simulink library "OpenSCENARIO"  (R2019a)
settings: Solver=VariableStepAuto  StartTime=0.0  StopTime=10.0  RelTol=1e-3
undefined symbols (not defined in the file or in its folder): A1, car, DiscIntNeverNeededParam, i, t1, W1
libraries: adeye_lib x6, $bdroot x2, simulink x2
settings Model: Creator=adeye  LastModifiedBy=adeye

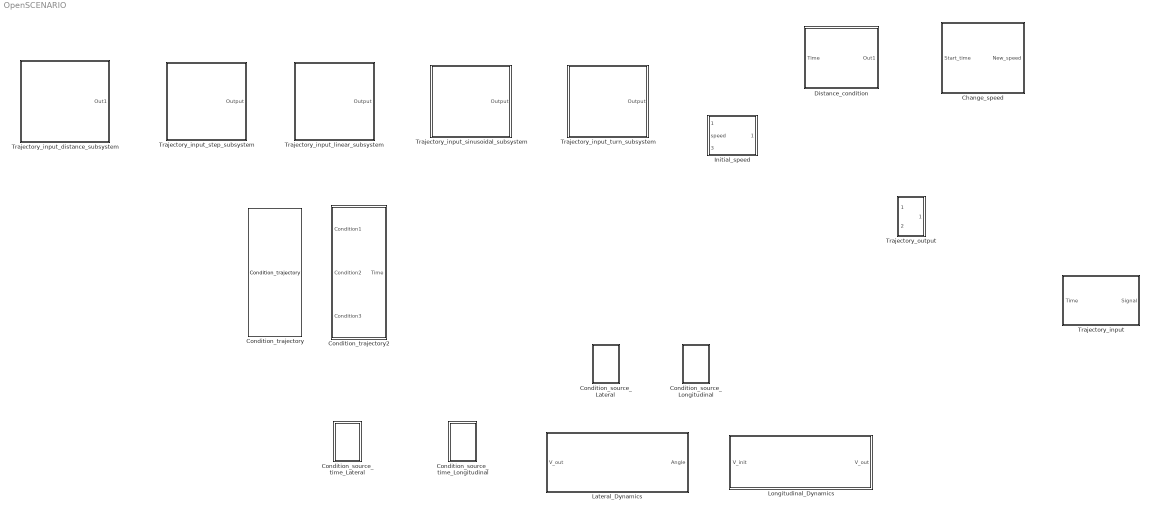
== system OpenSCENARIO ==
  Change_speed : Subsystem
  Condition_source_Lateral : Subsystem
  Condition_source_Longitudinal : Subsystem
  Condition_source_time_Lateral : Subsystem
  Condition_source_time_Longitudinal : Subsystem
  Condition_trajectory : $bdroot/Trajectory_input_step_subsystem/Condition_trajectory  SystemSampleTime=-1
      link override Gain2: Gain=1
      link override Switch1: Threshold=0.001
  Condition_trajectory2 : Subsystem
  Distance_condition : Subsystem
  Initial_speed : Subsystem
  Lateral_Dynamics : Subsystem
  Longitudinal_Dynamics : Subsystem
  Trajectory_input : Subsystem
  Trajectory_input_distance_subsystem : Subsystem
  Trajectory_input_linear_subsystem : Subsystem
  Trajectory_input_sinusoidal_subsystem : Subsystem
  Trajectory_input_step_subsystem : Subsystem
  Trajectory_input_turn_subsystem : Subsystem  AncestorBlock=OpenSCENARIO/Trajectory_input_sinusoidal_subsystem
  Trajectory_output : Subsystem

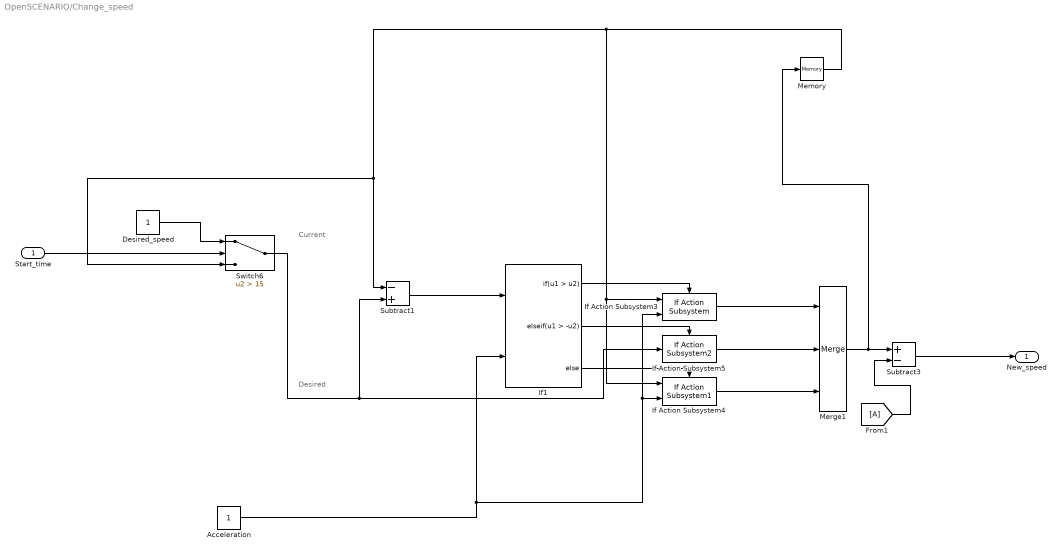
== system OpenSCENARIO/Change_speed ==
  note: Current
  note: Desired
  Start_time : Inport
  Acceleration : Constant
  Desired_speed : Constant
  If Action Subsystem3 : adeye_lib/Subsystem1/Subsystem/If Action Subsystem  SystemSampleTime=-1
  If Action Subsystem4 : adeye_lib/Subsystem1/Subsystem/If Action Subsystem1  SystemSampleTime=-1
  If Action Subsystem5 : adeye_lib/Subsystem1/Subsystem/If Action Subsystem2  SystemSampleTime=-1
  If1 : If  NumInputs=2  IfExpression=u1 > u2  ElseIfExpressions=u1 > -u2
  Memory : Memory  InitialCondition=-5/3.6
  Merge1 : Merge  Inputs=3
  Subtract1 : Sum  Inputs=-+
  Subtract3 : Sum  Inputs=+-
  Switch6 : Switch  Criteria=u2 > Threshold  Threshold=15
  "New_speed " : Outport
  wires:
  If Action Subsystem3/1 -> Merge1/1
  If Action Subsystem4/1 -> Merge1/3
  If1/1 -> If Action Subsystem3/Action
  Start_time/1 -> Switch6/2
  If Action Subsystem5/1 -> Merge1/2
  Acceleration/1 -> If1/2, If Action Subsystem4/2, If Action Subsystem3/2
  If1/3 -> If Action Subsystem4/Action
  If1/2 -> If Action Subsystem5/Action
  Desired_speed/1 -> Switch6/1
  Switch6/1 -> Subtract1/2, If Action Subsystem5/1
  Subtract1/1 -> If1/1
  Merge1/1 -> Memory/1, Subtract3/1
  [A] -> Subtract3/2
  Subtract3/1 -> "New_speed "/1
  Memory/1 -> If Action Subsystem3/1, If Action Subsystem4/1, Switch6/3, Subtract1/1

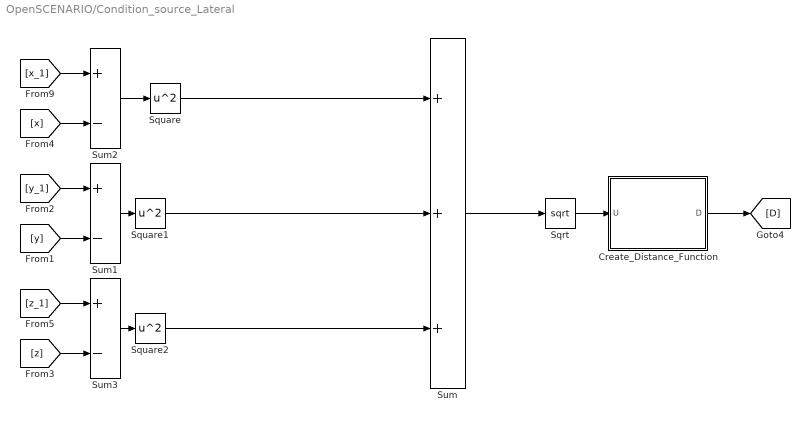
== system OpenSCENARIO/Condition_source_Lateral ==
  Create_Distance_Function : Subsystem
  Sqrt : Sqrt  SaturateOnIntegerOverflow=on
  Square : Math  Operator=square  SaturateOnIntegerOverflow=on
  Square1 : Math  Operator=square  SaturateOnIntegerOverflow=on
  Square2 : Math  Operator=square  SaturateOnIntegerOverflow=on
  Sum : Sum  Inputs=+++
  Sum1 : Sum  Inputs=+-
  Sum2 : Sum  Inputs=+-
  Sum3 : Sum  Inputs=+-
  wires:
  [x_1] -> Sum2/1
  [x] -> Sum2/2
  [y_1] -> Sum1/1
  [y] -> Sum1/2
  [z] -> Sum3/2
  [z_1] -> Sum3/1
  Sum/1 -> Sqrt/1
  Sum1/1 -> Square1/1
  Sum2/1 -> Square/1
  Square1/1 -> Sum/2
  Sum3/1 -> Square2/1
  Square2/1 -> Sum/3
  Square/1 -> Sum/1
  Create_Distance_Function/1(D) -> [D]
  Sqrt/1 -> Create_Distance_Function/1(U)

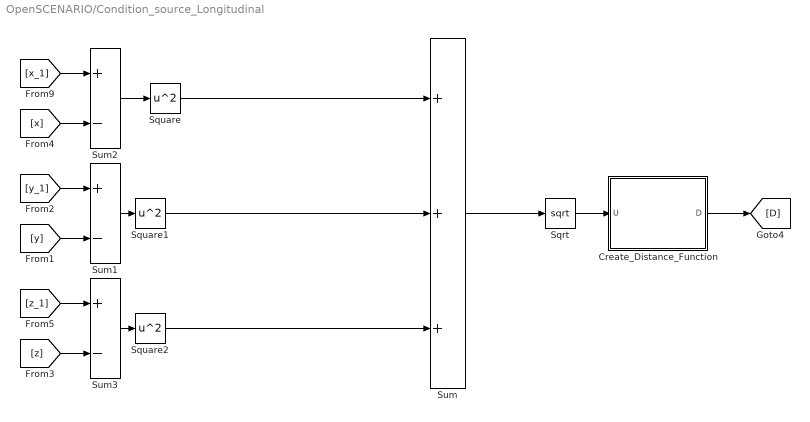
== system OpenSCENARIO/Condition_source_Longitudinal ==
  Create_Distance_Function : Subsystem
  Sqrt : Sqrt  SaturateOnIntegerOverflow=on
  Square : Math  Operator=square  SaturateOnIntegerOverflow=on
  Square1 : Math  Operator=square  SaturateOnIntegerOverflow=on
  Square2 : Math  Operator=square  SaturateOnIntegerOverflow=on
  Sum : Sum  Inputs=+++
  Sum1 : Sum  Inputs=+-
  Sum2 : Sum  Inputs=+-
  Sum3 : Sum  Inputs=+-
  wires:
  [x_1] -> Sum2/1
  [x] -> Sum2/2
  [y_1] -> Sum1/1
  [y] -> Sum1/2
  [z] -> Sum3/2
  [z_1] -> Sum3/1
  Sum/1 -> Sqrt/1
  Sum1/1 -> Square1/1
  Sum2/1 -> Square/1
  Square1/1 -> Sum/2
  Sum3/1 -> Square2/1
  Square2/1 -> Sum/3
  Square/1 -> Sum/1
  Create_Distance_Function/1(D) -> [D]
  Sqrt/1 -> Create_Distance_Function/1(U)

== system OpenSCENARIO/Condition_source_time_Lateral ==
  Constant : Constant
  Integrator : Integrator
  wires:
  Constant/1 -> Integrator/1
  Integrator/1 -> [D]

== system OpenSCENARIO/Condition_source_time_Longitudinal ==
  Constant : Constant
  Integrator : Integrator
  wires:
  Constant/1 -> Integrator/1
  Integrator/1 -> [D]

== system OpenSCENARIO/Condition_trajectory2 ==
  Condition1 : Inport
  Condition2 : Inport  Port=2
  Condition3 : Inport  Port=3
  Constant1 : Constant  Value=0
  Integrator1 : Integrator
  Rounding Function : Rounding
  Scope4 : Scope
  Switch1 : Switch  Criteria=u2 > Threshold  Threshold=-str2double(car(2).trajectory(1,i).condition.general.value)
  Variable Integer Delay : Delay  DelayLengthSource=Input port
      settings: InputPortMap=u0,p1
  Time : Outport
  wires:
  Switch1/1 -> Integrator1/1
  Condition2/1 -> Switch1/2
  Integrator1/1 -> Variable Integer Delay/1
  Variable Integer Delay/1 -> Scope4/1, Time/1
  Constant1/1 -> Rounding Function/1
  Rounding Function/1 -> Variable Integer Delay/2
  Condition1/1 -> Switch1/1
  Condition3/1 -> Switch1/3

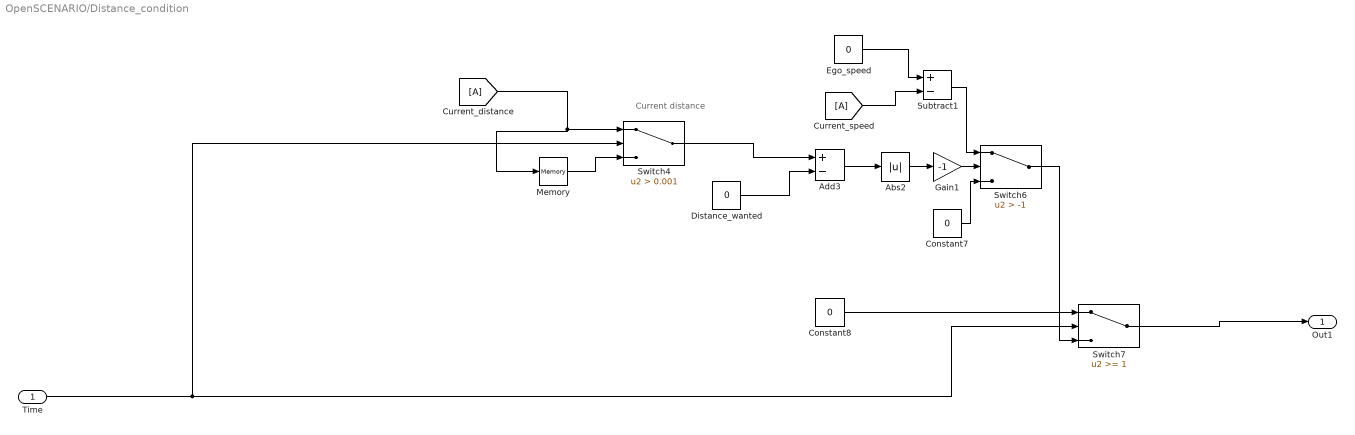
== system OpenSCENARIO/Distance_condition ==
  note: Current distance
  Time : Inport
  Abs2 : Abs  OutDataTypeStr=Inherit: Inherit via internal rule
  Add3 : Sum  Inputs=+-
  Constant7 : Constant  Value=0
  Constant8 : Constant  Value=0
  Distance_wanted : Constant  Value=0
  Ego_speed : Constant  Value=0
  Gain1 : Gain  Gain=-1
  Memory : Memory
  Subtract1 : Sum  Inputs=+-
  Switch4 : Switch  Criteria=u2 > Threshold  Threshold=0.001
  Switch6 : Switch  Criteria=u2 > Threshold  Threshold=-1
  Switch7 : Switch  Threshold=1
  Out1 : Outport
  wires:
  Gain1/1 -> Switch6/2
  Abs2/1 -> Gain1/1
  Switch7/1 -> Out1/1
  Constant8/1 -> Switch7/1
  Time/1 -> Switch4/2, Switch7/2
  Switch4/1 -> Add3/1
  [A] -> Subtract1/2
  Switch6/1 -> Switch7/3
  Constant7/1 -> Switch6/3
  Subtract1/1 -> Switch6/1
  Distance_wanted/1 -> Add3/2
  Ego_speed/1 -> Subtract1/1
  Add3/1 -> Abs2/1
  Memory/1 -> Switch4/3
  [A] -> Memory/1, Switch4/1

== system OpenSCENARIO/Initial_speed ==
  Initial_speed : Inport
  speed : Inport  Port=2
  Step_time : Inport  Port=3
  Clock : Clock
  If : If  NumInputs=2  IfExpression=u1 < u2
  If Action Subsystem : Subsystem  TreatAsAtomicUnit=on
  If Action Subsystem1 : Subsystem  TreatAsAtomicUnit=on
  Merge : Merge
  ego_speed : Outport
  wires:
  Initial_speed/1 -> If Action Subsystem/1(In1)
  Merge/1 -> ego_speed/1
  Clock/1 -> If/1
  If/1 -> If Action Subsystem/Action
  speed/1 -> If Action Subsystem1/1(In1)
  If/2 -> If Action Subsystem1/Action
  If Action Subsystem/1(Out1) -> Merge/1
  If Action Subsystem1/1(Out1) -> Merge/2
  Step_time/1 -> If/2

== system OpenSCENARIO/Lateral_Dynamics ==
  V_out : Inport
  Add : Sum
  Trajectory_output : Subsystem
  Angle : Outport
  tag scope: V_out=global
  wires:
  Trajectory_output/1(Angle) -> Angle/1
  Add/1 -> Trajectory_output/2(Signal)
  V_out/1 -> [V_out], Trajectory_output/1(V_init)

== system OpenSCENARIO/Longitudinal_Dynamics ==
  V_init : Inport
  Add : Sum
  V_out : Outport
  tag scope: V_in=global
  wires:
  Add/1 -> V_out/1
  V_init/1 -> [V_in], Add/1

== system OpenSCENARIO/Trajectory_input ==
  Time : Inport
  Constant3 : Constant  Value=A1
  Gain4 : Gain  Gain=-1
  Gain5 : Gain  Gain=A1
  Gain6 : Gain  Gain=W1
  Memory : Memory
  Sine1 : Trigonometry
  Switch3 : Switch  Criteria=u2 > Threshold  Threshold=-t1
  Signal : Outport
  wires:
  Time/1 -> Gain5/1, Gain4/1, Gain6/1
  Gain6/1 -> Sine1/1
  Gain4/1 -> Switch3/2
  Switch3/1 -> Memory/1, Signal/1
  Gain5/1 -> Switch3/1
  Memory/1 -> Switch3/3

== system OpenSCENARIO/Trajectory_input_distance_subsystem ==
  Condition_trajectory : $bdroot/Trajectory_input_step_subsystem/Condition_trajectory  SystemSampleTime=-1
      link override Gain2: Gain=1
      link override Switch1: Threshold=0.001
      link override Switch2: Threshold=0  Criteria=u2 >= Threshold
  Distance_condition : Subsystem  AncestorBlock=OpenSCENARIO/Distance_condition
  Out1 : Outport
  wires:
  Condition_trajectory/1 -> Distance_condition/1(Time)
  Distance_condition/1(Out1) -> Out1/1

== system OpenSCENARIO/Trajectory_input_linear_subsystem ==
  Change_speed : Subsystem  AncestorBlock=OpenSCENARIO/Change_speed
  Condition_trajectory : Subsystem
  Output : Outport
  wires:
  Change_speed/1("New_speed ") -> Output/1
  Condition_trajectory/1(Time) -> Change_speed/1(Start_time)

== system OpenSCENARIO/Trajectory_input_sinusoidal_subsystem ==
  Condition_trajectory : Subsystem
  Trajectory_input : Subsystem
  Output : Outport
  wires:
  Condition_trajectory/1(Time) -> Trajectory_input/1(Time)
  Trajectory_input/1(Signal) -> Output/1

== system OpenSCENARIO/Trajectory_input_step_subsystem ==
  Condition_trajectory : Subsystem
  Trajectory_input : Subsystem
  Output : Outport
  wires:
  Condition_trajectory/1(Time) -> Trajectory_input/1(Time)
  Trajectory_input/1(Signal) -> Output/1

== system OpenSCENARIO/Trajectory_input_turn_subsystem ==
  Condition_trajectory : Subsystem
  Trajectory_input : Subsystem
  Output : Outport
  wires:
  Condition_trajectory/1(Time) -> Trajectory_input/1(Time)
  Trajectory_input/1(Signal) -> Output/1

== system OpenSCENARIO/Trajectory_output ==
  V_init : Inport
  Signal : Inport  Port=2
  Asin : Trigonometry  Operator=asin
  Discrete Derivative : simulink/Discrete/Discrete Derivative  gainval=1.0  ICPrevScaledInput=0.0  OutMin=[]  OutMax=[]  OutDataType=fixdt(1, 16)  OutScaling=2^-10  DoSatur=off
  Divide : Product  Inputs=/*
  Angle : Outport
  wires:
  Divide/1 -> Asin/1
  Discrete Derivative/1 -> Divide/2
  Signal/1 -> Discrete Derivative/1
  V_init/1 -> Divide/1
  Asin/1 -> Angle/1

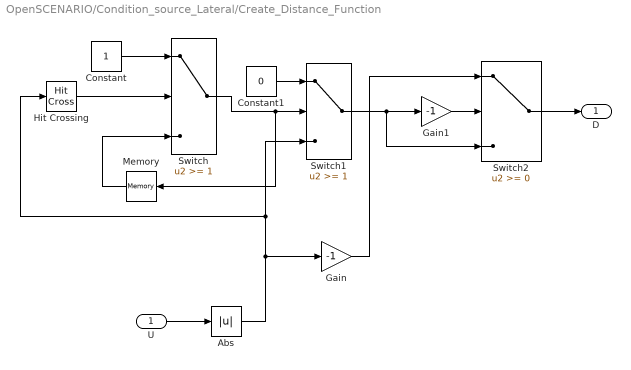
== system OpenSCENARIO/Condition_source_Lateral/Create_Distance_Function ==
  U : Inport
  Abs : Abs
  Constant : Constant
  Constant1 : Constant  Value=0
  Gain : Gain  Gain=-1
  Gain1 : Gain  Gain=-1
  Hit Crossing : HitCross  HitCrossingOffset=0.5
  Memory : Memory
  Switch : Switch  Threshold=1
  Switch1 : Switch  Threshold=1
  Switch2 : Switch
  D : Outport
  wires:
  Abs/1 -> Switch1/3, Hit Crossing/1, Gain/1
  Constant1/1 -> Switch1/1
  Memory/1 -> Switch/3
  Switch/1 -> Memory/1, Switch1/2
  Gain1/1 -> Switch2/2
  Hit Crossing/1 -> Switch/2
  Switch1/1 -> Switch2/3, Gain1/1
  Switch2/1 -> D/1
  Gain/1 -> Switch2/1
  Constant/1 -> Switch/1
  U/1 -> Abs/1

== system OpenSCENARIO/Condition_source_Longitudinal/Create_Distance_Function ==
  U : Inport
  Abs : Abs
  Constant : Constant
  Constant1 : Constant  Value=0
  Gain : Gain  Gain=-1
  Gain1 : Gain  Gain=-1
  Hit Crossing : HitCross  HitCrossingOffset=0.5
  Memory : Memory
  Switch : Switch  Threshold=1
  Switch1 : Switch  Threshold=1
  Switch2 : Switch
  D : Outport
  wires:
  Abs/1 -> Switch1/3, Hit Crossing/1, Gain/1
  Constant1/1 -> Switch1/1
  Memory/1 -> Switch/3
  Switch/1 -> Memory/1, Switch1/2
  Gain1/1 -> Switch2/2
  Hit Crossing/1 -> Switch/2
  Switch1/1 -> Switch2/3, Gain1/1
  Switch2/1 -> D/1
  Gain/1 -> Switch2/1
  Constant/1 -> Switch/1
  U/1 -> Abs/1

== system OpenSCENARIO/Initial_speed/If Action Subsystem ==
  In1 : Inport
  Action Port : ActionPort
  Out1 : Outport
  wires:
  In1/1 -> Out1/1

== system OpenSCENARIO/Initial_speed/If Action Subsystem1 ==
  In1 : Inport
  Action Port : ActionPort
  Out1 : Outport
  wires:
  In1/1 -> Out1/1

== system OpenSCENARIO/Lateral_Dynamics/Trajectory_output ==
  V_init : Inport
  Signal : Inport  Port=2
  Asin : Trigonometry  Operator=asin
  Constant : Constant
  Discrete Derivative : simulink/Discrete/Discrete Derivative  gainval=1.0  ICPrevScaledInput=0.0  OutMin=[]  OutMax=[]  OutDataType=fixdt(1, 16)  OutScaling=2^-10  DoSatur=off
  Divide : Product  Inputs=/*
  Switch : Switch  Criteria=u2 > Threshold
  Angle : Outport
  wires:
  Divide/1 -> Asin/1
  Discrete Derivative/1 -> Divide/2
  Signal/1 -> Discrete Derivative/1
  V_init/1 -> Divide/1
  Switch/1 -> Angle/1
  Asin/1 -> Switch/1
  [W] -> Switch/2
  Constant/1 -> Switch/3

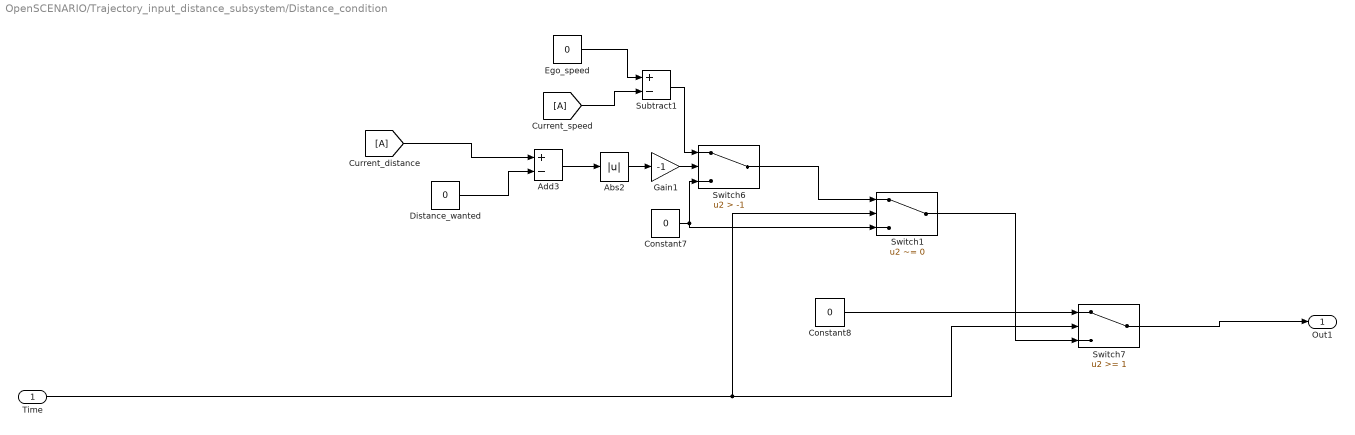
== system OpenSCENARIO/Trajectory_input_distance_subsystem/Distance_condition ==
  Time : Inport
  Abs2 : Abs  OutDataTypeStr=Inherit: Inherit via internal rule
  Add3 : Sum  Inputs=+-
  Constant7 : Constant  Value=0
  Constant8 : Constant  Value=0
  Distance_wanted : Constant  Value=0
  Ego_speed : Constant  Value=0
  Gain1 : Gain  Gain=-1
  Subtract1 : Sum  Inputs=+-
  Switch1 : Switch  Criteria=u2 ~= 0  Threshold=-1
  Switch6 : Switch  Criteria=u2 > Threshold  Threshold=-1
  Switch7 : Switch  Threshold=1
  Out1 : Outport
  wires:
  Gain1/1 -> Switch6/2
  Abs2/1 -> Gain1/1
  Switch7/1 -> Out1/1
  Constant8/1 -> Switch7/1
  Time/1 -> Switch1/2, Switch7/2
  [A] -> Add3/1
  [A] -> Subtract1/2
  Constant7/1 -> Switch6/3, Switch1/3
  Subtract1/1 -> Switch6/1
  Distance_wanted/1 -> Add3/2
  Ego_speed/1 -> Subtract1/1
  Add3/1 -> Abs2/1
  Switch1/1 -> Switch7/3
  Switch6/1 -> Switch1/1

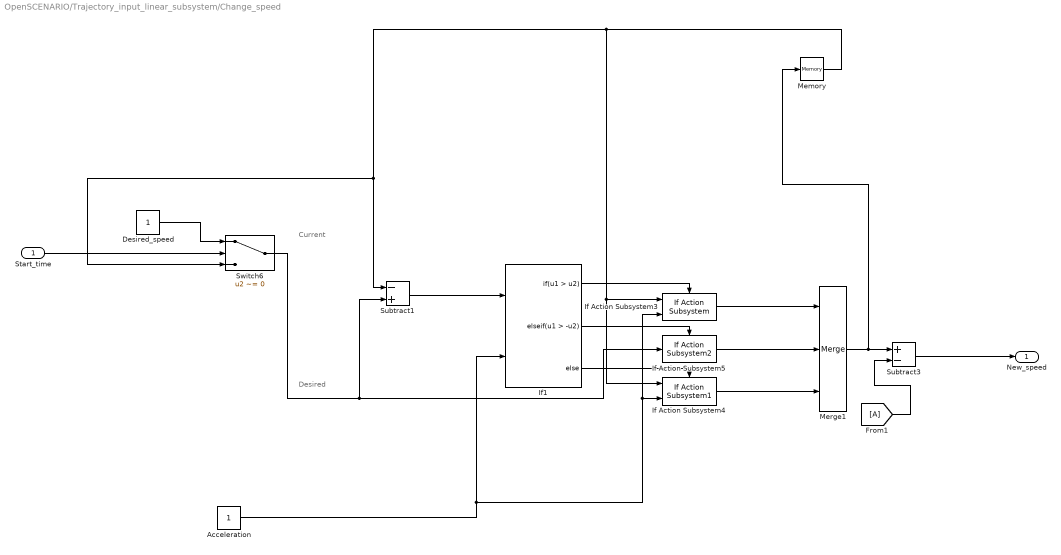
== system OpenSCENARIO/Trajectory_input_linear_subsystem/Change_speed ==
  note: Desired
  note: Current
  Start_time : Inport
  Acceleration : Constant
  Desired_speed : Constant
  If Action Subsystem3 : adeye_lib/Subsystem1/Subsystem/If Action Subsystem  SystemSampleTime=-1
  If Action Subsystem4 : adeye_lib/Subsystem1/Subsystem/If Action Subsystem1  SystemSampleTime=-1
  If Action Subsystem5 : adeye_lib/Subsystem1/Subsystem/If Action Subsystem2  SystemSampleTime=-1
  If1 : If  NumInputs=2  IfExpression=u1 > u2  ElseIfExpressions=u1 > -u2
  Memory : Memory  InitialCondition=-5/3.6
  Merge1 : Merge  Inputs=3
  Subtract1 : Sum  Inputs=-+
  Subtract3 : Sum  Inputs=+-
  Switch6 : Switch  Criteria=u2 ~= 0  Threshold=15
  "New_speed " : Outport
  wires:
  Memory/1 -> Subtract1/1, Switch6/3, If Action Subsystem4/1, If Action Subsystem3/1
  Subtract3/1 -> "New_speed "/1
  [A] -> Subtract3/2
  Merge1/1 -> Subtract3/1, Memory/1
  Subtract1/1 -> If1/1
  Switch6/1 -> If Action Subsystem5/1, Subtract1/2
  Desired_speed/1 -> Switch6/1
  If1/2 -> If Action Subsystem5/Action
  If1/3 -> If Action Subsystem4/Action
  Acceleration/1 -> If Action Subsystem3/2, If Action Subsystem4/2, If1/2
  If Action Subsystem5/1 -> Merge1/2
  Start_time/1 -> Switch6/2
  If1/1 -> If Action Subsystem3/Action
  If Action Subsystem4/1 -> Merge1/3
  If Action Subsystem3/1 -> Merge1/1

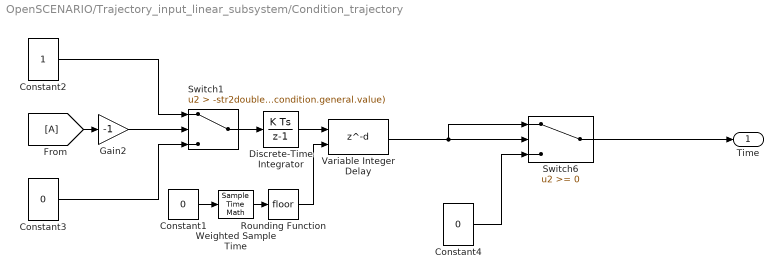
== system OpenSCENARIO/Trajectory_input_linear_subsystem/Condition_trajectory ==
  Constant1 : Constant  Value=0
  Constant2 : Constant
  Constant3 : Constant  Value=0
  Constant4 : Constant  Value=0
  Discrete-Time Integrator : DiscreteIntegrator  SampleTime=-1  ICPrevOutput=DiscIntNeverNeededParam  ICPrevScaledInput=DiscIntNeverNeededParam
  Gain2 : Gain  Gain=-1
  Rounding Function : Rounding
  Switch1 : Switch  Criteria=u2 > Threshold  Threshold=-str2double(car(2).trajectory(1,i).condition.general.value)
  Switch6 : Switch
  Variable Integer Delay : Delay  DelayLengthSource=Input port  DelayLengthUpperLimit=999
      settings: InputPortMap=u0,p1
  Weighted Sample Time : SampleTimeMath  TsampMathOp=/  TsampMathImp=Offline Scaling Adjustment
  Time : Outport
  wires:
  Rounding Function/1 -> Variable Integer Delay/2
  Constant1/1 -> Weighted Sample Time/1
  Discrete-Time Integrator/1 -> Variable Integer Delay/1
  Gain2/1 -> Switch1/2
  Switch1/1 -> Discrete-Time Integrator/1
  Constant3/1 -> Switch1/3
  Constant2/1 -> Switch1/1
  [A] -> Gain2/1
  Weighted Sample Time/1 -> Rounding Function/1
  Switch6/1 -> Time/1
  Variable Integer Delay/1 -> Switch6/1, Switch6/2
  Constant4/1 -> Switch6/3

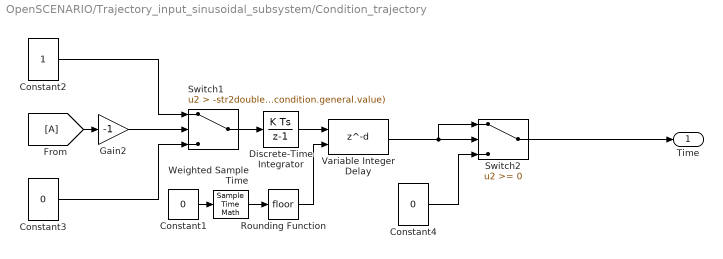
== system OpenSCENARIO/Trajectory_input_sinusoidal_subsystem/Condition_trajectory ==
  Constant1 : Constant  Value=0
  Constant2 : Constant
  Constant3 : Constant  Value=0
  Constant4 : Constant  Value=0
  Discrete-Time Integrator : DiscreteIntegrator  SampleTime=-1  ICPrevOutput=DiscIntNeverNeededParam  ICPrevScaledInput=DiscIntNeverNeededParam
  Gain2 : Gain  Gain=-1
  Rounding Function : Rounding
  Switch1 : Switch  Criteria=u2 > Threshold  Threshold=-str2double(car(2).trajectory(1,i).condition.general.value)
  Switch2 : Switch
  Variable Integer Delay : Delay  DelayLengthSource=Input port  DelayLengthUpperLimit=999
      settings: InputPortMap=u0,p1
  Weighted Sample Time : SampleTimeMath  TsampMathOp=/  TsampMathImp=Offline Scaling Adjustment
  Time : Outport
  wires:
  Rounding Function/1 -> Variable Integer Delay/2
  Discrete-Time Integrator/1 -> Variable Integer Delay/1
  Gain2/1 -> Switch1/2
  Switch1/1 -> Discrete-Time Integrator/1
  Constant3/1 -> Switch1/3
  Constant2/1 -> Switch1/1
  [A] -> Gain2/1
  Constant1/1 -> Weighted Sample Time/1
  Weighted Sample Time/1 -> Rounding Function/1
  Switch2/1 -> Time/1
  Variable Integer Delay/1 -> Switch2/1, Switch2/2
  Constant4/1 -> Switch2/3

== system OpenSCENARIO/Trajectory_input_sinusoidal_subsystem/Trajectory_input ==
  Time : Inport
  Constant3 : Constant  Value=A1
  Cos : Trigonometry  Operator=cos
  Gain4 : Gain  Gain=-1
  Gain5 : Gain  Gain=A1
  Gain6 : Gain  Gain=W1
  Switch3 : Switch  Criteria=u2 > Threshold  Threshold=-t1
  Signal : Outport
  tag scope: W=global
  wires:
  Gain5/1 -> Switch3/1
  Constant3/1 -> Switch3/3
  Time/1 -> Gain4/1, Gain6/1
  Gain6/1 -> Cos/1
  Gain4/1 -> [W], Switch3/2
  Cos/1 -> Gain5/1
  Switch3/1 -> Signal/1

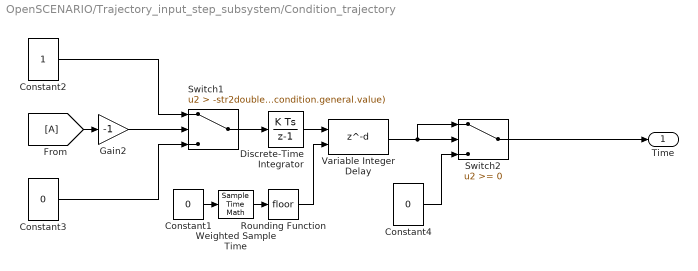
== system OpenSCENARIO/Trajectory_input_step_subsystem/Condition_trajectory ==
  Constant1 : Constant  Value=0
  Constant2 : Constant
  Constant3 : Constant  Value=0
  Constant4 : Constant  Value=0
  Discrete-Time Integrator : DiscreteIntegrator  SampleTime=-1  ICPrevOutput=DiscIntNeverNeededParam  ICPrevScaledInput=DiscIntNeverNeededParam
  Gain2 : Gain  Gain=-1
  Rounding Function : Rounding
  Switch1 : Switch  Criteria=u2 > Threshold  Threshold=-str2double(car(2).trajectory(1,i).condition.general.value)
  Switch2 : Switch
  Variable Integer Delay : Delay  DelayLengthSource=Input port  DelayLengthUpperLimit=999
      settings: InputPortMap=u0,p1
  Weighted Sample Time : SampleTimeMath  TsampMathOp=/  TsampMathImp=Offline Scaling Adjustment
  Time : Outport
  wires:
  Rounding Function/1 -> Variable Integer Delay/2
  Discrete-Time Integrator/1 -> Variable Integer Delay/1
  Gain2/1 -> Switch1/2
  Switch1/1 -> Discrete-Time Integrator/1
  Constant3/1 -> Switch1/3
  Constant2/1 -> Switch1/1
  [A] -> Gain2/1
  Weighted Sample Time/1 -> Rounding Function/1
  Constant1/1 -> Weighted Sample Time/1
  Switch2/1 -> Time/1
  Variable Integer Delay/1 -> Switch2/1, Switch2/2
  Constant4/1 -> Switch2/3

== system OpenSCENARIO/Trajectory_input_step_subsystem/Trajectory_input ==
  Time : Inport
  Constant2 : Constant  Value=0
  Switch1 : Switch  Criteria=u2 ~= 0  Threshold=0.000001
  speed : Constant
  Signal : Outport
  wires:
  Constant2/1 -> Switch1/3
  Time/1 -> Switch1/2
  speed/1 -> Switch1/1
  Switch1/1 -> Signal/1

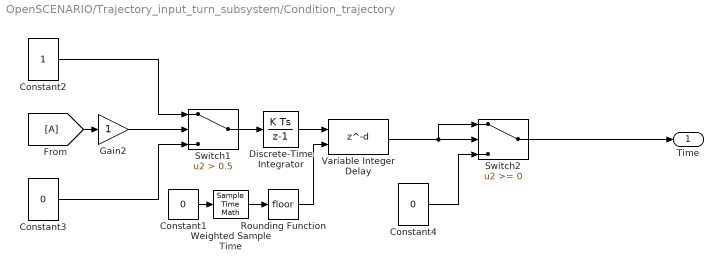
== system OpenSCENARIO/Trajectory_input_turn_subsystem/Condition_trajectory ==
  Constant1 : Constant  Value=0
  Constant2 : Constant
  Constant3 : Constant  Value=0
  Constant4 : Constant  Value=0
  Discrete-Time Integrator : DiscreteIntegrator  SampleTime=-1  ICPrevOutput=DiscIntNeverNeededParam  ICPrevScaledInput=DiscIntNeverNeededParam
  Gain2 : Gain
  Rounding Function : Rounding
  Switch1 : Switch  Criteria=u2 > Threshold  Threshold=0.5
  Switch2 : Switch
  Variable Integer Delay : Delay  DelayLengthSource=Input port  DelayLengthUpperLimit=999
      settings: InputPortMap=u0,p1
  Weighted Sample Time : SampleTimeMath  TsampMathOp=/  TsampMathImp=Offline Scaling Adjustment
  Time : Outport
  wires:
  Rounding Function/1 -> Variable Integer Delay/2
  Discrete-Time Integrator/1 -> Variable Integer Delay/1
  Gain2/1 -> Switch1/2
  Switch1/1 -> Discrete-Time Integrator/1
  Constant3/1 -> Switch1/3
  Constant2/1 -> Switch1/1
  [A] -> Gain2/1
  Constant1/1 -> Weighted Sample Time/1
  Weighted Sample Time/1 -> Rounding Function/1
  Switch2/1 -> Time/1
  Variable Integer Delay/1 -> Switch2/1, Switch2/2
  Constant4/1 -> Switch2/3

== system OpenSCENARIO/Trajectory_input_turn_subsystem/Trajectory_input ==
  Time : Inport
  Constant3 : Constant  Value=A1
  Cos : Trigonometry  Operator=cos
  Gain4 : Gain  Gain=-1
  Gain5 : Gain  Gain=A1
  Gain6 : Gain  Gain=W1
  Switch3 : Switch  Criteria=u2 > Threshold  Threshold=-t1
  Signal : Outport
  tag scope: W=global
  wires:
  Gain5/1 -> Switch3/1
  Constant3/1 -> Switch3/3
  Time/1 -> Gain4/1, Gain6/1
  Gain6/1 -> Cos/1
  Gain4/1 -> [W], Switch3/2
  Cos/1 -> Gain5/1
  Switch3/1 -> Signal/1
